simulink model "firstSimulink"  (R2023a)
settings: Solver=VariableStepAuto  StartTime=0.0  StopTime=50  RelTol=1e-3
settings Model: Creator=z'k'x  LastModifiedBy=z'k'x

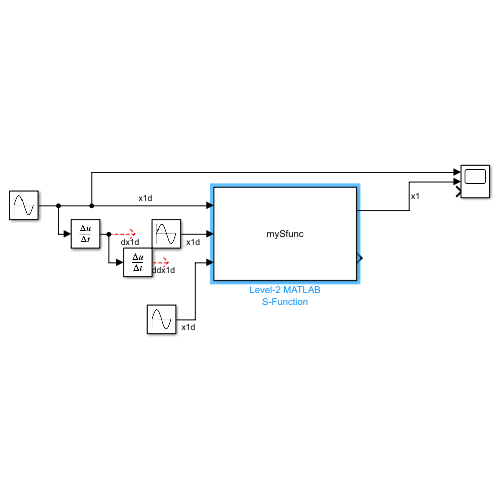
[thumbnail: Simulink's stored preview of the top-level diagram]
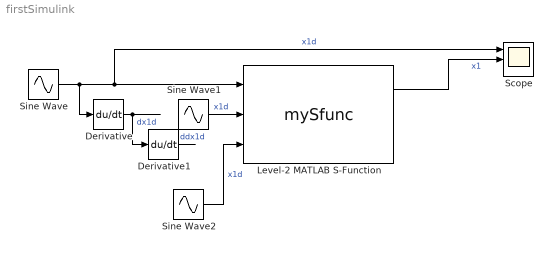
== system firstSimulink ==
  Derivative : Derivative
  Derivative1 : Derivative
  Level-2 MATLAB S-Function : M-S-Function  FunctionName=mySfunc
  Scope : Scope  NumInputPorts=3
  Sine Wave : Sin  SampleTime=0
  Sine Wave1 : Sin  Phase=pi/2  SampleTime=0
  Sine Wave2 : Sin  Phase=pi  SampleTime=0
  wires:
  Level-2 MATLAB S-Function/1 -> Scope/2  "x1"
  Sine Wave/1 -> Derivative/1, Level-2 MATLAB S-Function/1, Scope/1  "x1d"
  Derivative/1 -> Derivative1/1  "dx1d"
  Derivative1/1 -> ?  "ddx1d"
  Sine Wave1/1 -> Level-2 MATLAB S-Function/2  "x1d"
  Sine Wave2/1 -> Level-2 MATLAB S-Function/3  "x1d"
